simulink model "Test3S150Board_Leds"  (Simulink 6.4)
settings: Solver=ode45  SolverMode=SingleTasking  StartTime=0.0  StopTime=100000.0  FixedStep=1  RelTol=1e-3
InitFcn:
  | %% DSPBuilder Start
  | alt_dspbuilder_update_model(bdroot)
  | %% DSPBuilder End
undefined symbols (not defined in the file): Pin_A19, Pin_A20, Pin_B19, Pin_C18, Pin_J19, Pin_K19, Pin_L19, Pin_L20
libraries: allblocks_alteradspbuilder2 x19, Stratix_III_EP3SL150_alteradspbuilder2 x14
settings Model: Creator=lkong  LastModifiedBy=lkong
settings DataIOCC: SignalLoggingName=sigsOut
settings OptimizationCC: InlineInvariantSignals=on
settings DebuggingCC: SolverPrmCheckMsg=none  StrictBusMsg=None
settings HardwareCC: TargetUnknown=on
settings GRTTargetCC: ModelReferenceCompliant=off  MatFileLogging=off

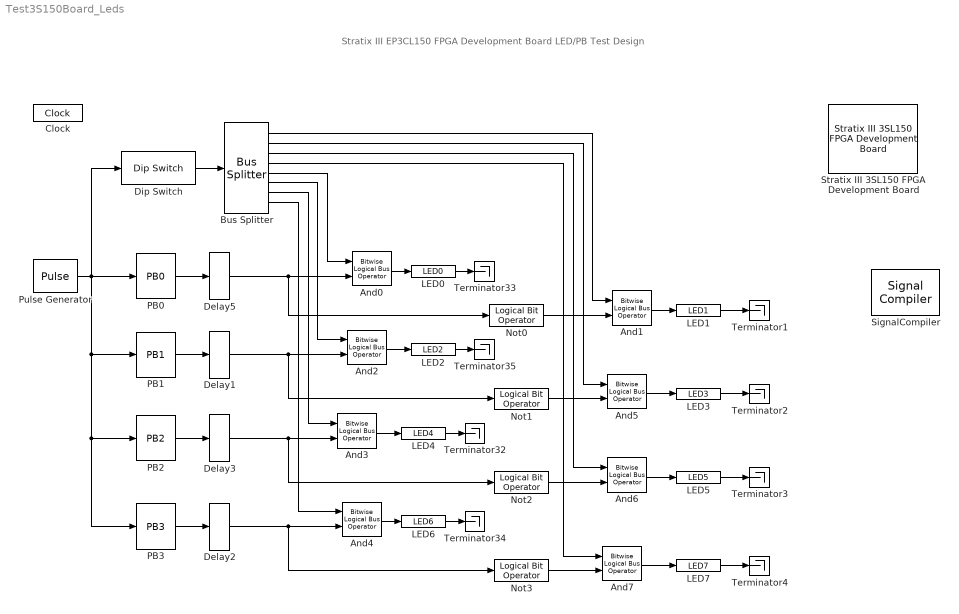
== system Test3S150Board_Leds ==
  note: Stratix III EP3CL150 FPGA Development Board LED/PB Test Design
  And{0..7} (8 alike) : allblocks_alteradspbuilder2/Bitwise Logical Bus Operator  BusType=Inferred  bwl=1  bwr=0  LogicalOperator=AND  pipeline_display=0
  Bus Splitter : allblocks_alteradspbuilder2/Bus Splitter  BusType=Signed Integer  bwl=8  bwr=0  pipeline_display=0
  Clock : allblocks_alteradspbuilder2/Clock  ClockPeriod=10  ClockPeriodUnit=ns  SampleTime=1  SimulationStartCycle=5  PhaseOffset=0  Reset=aclr  ResetType=Active Low  Export=off
  Delay1 : allblocks_alteradspbuilder2/Delay  pipeline=1  pipeline_display=1  ClockPhase=1  use_ena=off  use_sclr=off  allowFloatingPointOverride=on  logOutputs=off  logFile=d:\ws80\workspace\documentation\designExamples\demos\board\stratixIII_DSPBoard_3S150\tb_Test3S150Board_Leds\Test3S150Board%5FLeds_Delay1.fixedpointlog  use_init=off  reset_value=1
  Delay2 : allblocks_alteradspbuilder2/Delay  pipeline=1  pipeline_display=1  ClockPhase=1  use_ena=off  use_sclr=off  allowFloatingPointOverride=on  logOutputs=off  logFile=d:\ws80\workspace\documentation\designExamples\demos\board\stratixIII_DSPBoard_3S150\tb_Test3S150Board_Leds\Test3S150Board%5FLeds_Delay2.fixedpointlog  use_init=off  reset_value=1
  Delay3 : allblocks_alteradspbuilder2/Delay  pipeline=1  pipeline_display=1  ClockPhase=1  use_ena=off  use_sclr=off  allowFloatingPointOverride=on  logOutputs=off  logFile=d:\ws80\workspace\documentation\designExamples\demos\board\stratixIII_DSPBoard_3S150\tb_Test3S150Board_Leds\Test3S150Board%5FLeds_Delay3.fixedpointlog  use_init=off  reset_value=1
  Delay5 : allblocks_alteradspbuilder2/Delay  pipeline=1  pipeline_display=1  ClockPhase=1  use_ena=off  use_sclr=off  allowFloatingPointOverride=on  logOutputs=off  logFile=d:\ws80\workspace\documentation\designExamples\demos\board\stratixIII_DSPBoard_3S150\tb_Test3S150Board_Leds\Test3S150Board%5FLeds_Delay5.fixedpointlog  use_init=off  reset_value=1
  Dip Switch : Stratix_III_EP3SL150_alteradspbuilder2/Dip Switch  iofile=d:\ws80\workspace\documentation\designExamples\demos\board\stratixIII_DSPBoard_3S150\tb_Test3S150Board_Leds\Test3S150Board%5FLeds_Dip+Switch.salt  externalType=Inferred  SpecifyClock=off  location=Pin_B19,Pin_A19,Pin_C18,Pin_A20,Pin_K19,Pin_J19,Pin_L19,Pin_L20
  LED0 : Stratix_III_EP3SL150_alteradspbuilder2/LED0  iofile=d:\ws80\workspace\documentation\designExamples\demos\board\stratixIII_DSPBoard_3S150\tb_Test3S150Board_Leds\Test3S150Board%5FLeds_LED0.capture  externalType=Inferred  location=Pin_F21
  LED1 : Stratix_III_EP3SL150_alteradspbuilder2/LED1  iofile=d:\ws80\workspace\documentation\designExamples\demos\board\stratixIII_DSPBoard_3S150\tb_Test3S150Board_Leds\Test3S150Board%5FLeds_LED1.capture  externalType=Inferred  location=Pin_C23
  LED2 : Stratix_III_EP3SL150_alteradspbuilder2/LED2  iofile=d:\ws80\workspace\documentation\designExamples\demos\board\stratixIII_DSPBoard_3S150\tb_Test3S150Board_Leds\Test3S150Board%5FLeds_LED2.capture  externalType=Inferred  location=Pin_B23
  LED3 : Stratix_III_EP3SL150_alteradspbuilder2/LED3  iofile=d:\ws80\workspace\documentation\designExamples\demos\board\stratixIII_DSPBoard_3S150\tb_Test3S150Board_Leds\Test3S150Board%5FLeds_LED3.capture  externalType=Inferred  location=Pin_A23
  LED4 : Stratix_III_EP3SL150_alteradspbuilder2/LED4  iofile=d:\ws80\workspace\documentation\designExamples\demos\board\stratixIII_DSPBoard_3S150\tb_Test3S150Board_Leds\Test3S150Board%5FLeds_LED4.capture  externalType=Inferred  location=Pin_D19
  LED5 : Stratix_III_EP3SL150_alteradspbuilder2/LED5  iofile=d:\ws80\workspace\documentation\designExamples\demos\board\stratixIII_DSPBoard_3S150\tb_Test3S150Board_Leds\Test3S150Board%5FLeds_LED5.capture  externalType=Inferred  location=Pin_C19
  LED6 : Stratix_III_EP3SL150_alteradspbuilder2/LED6  iofile=d:\ws80\workspace\documentation\designExamples\demos\board\stratixIII_DSPBoard_3S150\tb_Test3S150Board_Leds\Test3S150Board%5FLeds_LED6.capture  externalType=Inferred  location=Pin_F19
  LED7 : Stratix_III_EP3SL150_alteradspbuilder2/LED7  iofile=d:\ws80\workspace\documentation\designExamples\demos\board\stratixIII_DSPBoard_3S150\tb_Test3S150Board_Leds\Test3S150Board%5FLeds_LED7.capture  externalType=Inferred  location=Pin_E19
  Not{0..3} (4 alike) : allblocks_alteradspbuilder2/Logical Bit Operator  LogicalOperator=NOT  user_inputs=2  pipeline_display=0
  PB0 : Stratix_III_EP3SL150_alteradspbuilder2/PB0  iofile=d:\ws80\workspace\documentation\designExamples\demos\board\stratixIII_DSPBoard_3S150\tb_Test3S150Board_Leds\Test3S150Board%5FLeds_PB0.salt  externalType=Inferred  SpecifyClock=off  location=Pin_B17
  PB1 : Stratix_III_EP3SL150_alteradspbuilder2/PB1  iofile=d:\ws80\workspace\documentation\designExamples\demos\board\stratixIII_DSPBoard_3S150\tb_Test3S150Board_Leds\Test3S150Board%5FLeds_PB1.salt  externalType=Inferred  SpecifyClock=off  location=Pin_A17
  PB2 : Stratix_III_EP3SL150_alteradspbuilder2/PB2  iofile=d:\ws80\workspace\documentation\designExamples\demos\board\stratixIII_DSPBoard_3S150\tb_Test3S150Board_Leds\Test3S150Board%5FLeds_PB2.salt  externalType=Inferred  SpecifyClock=off  location=Pin_A16
  PB3 : Stratix_III_EP3SL150_alteradspbuilder2/PB3  iofile=d:\ws80\workspace\documentation\designExamples\demos\board\stratixIII_DSPBoard_3S150\tb_Test3S150Board_Leds\Test3S150Board%5FLeds_PB3.salt  externalType=Inferred  SpecifyClock=off  location=Pin_K17
  Pulse Generator : DiscretePulseGenerator  Period=20000  PulseWidth=2
  SignalCompiler : allblocks_alteradspbuilder2/Signal Compiler  DeviceFamily=Stratix III  DeviceName=EP3SL150F1152C4ES  EnableSignalTap=on  SignalTapDepth=512  UseBoardBlock=on  StpUseDefaultClock=on  StpClock=Clock  ExportDir=D:\MATLAB\R2006a\work
  "Stratix III 3SL150 FPGA Development Board " : Stratix_III_EP3SL150_alteradspbuilder2/Stratix III 3SL150 FPGA Development Board   ClockPinIn=Pin_T33  GlobalResetPin=PIN_AP5  device=EP3SL150F1152C4ES
  Terminator{1..4,32..35} (8 alike) : Terminator
  wires:
  PB0/1 -> Delay5/1
  PB1/1 -> Delay1/1
  PB2/1 -> Delay3/1
  PB3/1 -> Delay2/1
  Delay2/1 -> Not3/1, And4/2
  Delay3/1 -> Not2/1, And3/2
  Delay1/1 -> Not1/1, And2/2
  Delay5/1 -> Not0/1, And0/2
  LED4/1 -> Terminator32/1
  LED0/1 -> Terminator33/1
  LED6/1 -> Terminator34/1
  LED2/1 -> Terminator35/1
  Pulse Generator/1 -> PB2/1, PB3/1, PB1/1, Dip Switch/1, PB0/1
  LED1/1 -> Terminator1/1
  LED3/1 -> Terminator2/1
  LED5/1 -> Terminator3/1
  LED7/1 -> Terminator4/1
  Dip Switch/1 -> Bus Splitter/1
  And0/1 -> LED0/1
  Not0/1 -> And1/2
  And1/1 -> LED1/1
  And2/1 -> LED2/1
  And3/1 -> LED4/1
  And4/1 -> LED6/1
  Bus Splitter/1 -> And1/1
  And5/1 -> LED3/1
  Not1/1 -> And5/2
  Bus Splitter/2 -> And5/1
  And6/1 -> LED5/1
  Not2/1 -> And6/2
  And7/1 -> LED7/1
  Bus Splitter/3 -> And6/1
  Bus Splitter/4 -> And7/1
  Not3/1 -> And7/2
  Bus Splitter/8 -> And4/1
  Bus Splitter/7 -> And3/1
  Bus Splitter/6 -> And2/1
  Bus Splitter/5 -> And0/1
